simulink model "FMCW_FPGA_Algorithm_Sim"  (R2026a)
settings: Solver=FixedStepDiscrete  StartTime=0  StopTime=simFpgaStopTime  FixedStep=simTs
undefined symbols (not defined in the file): simTemperatureSetpointC, simTs
settings Model: Creator=Administrator  LastModifiedBy=Administrator

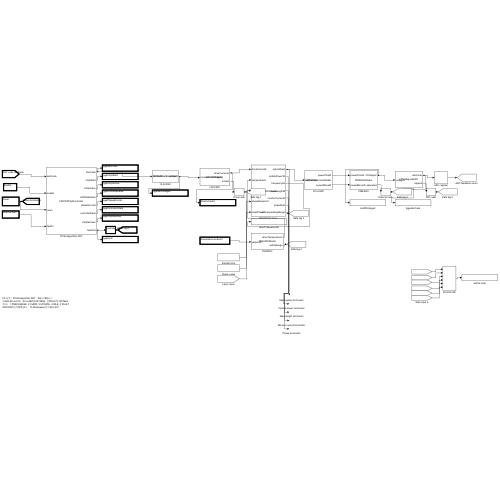
[thumbnail: Simulink's stored preview of the top-level diagram]
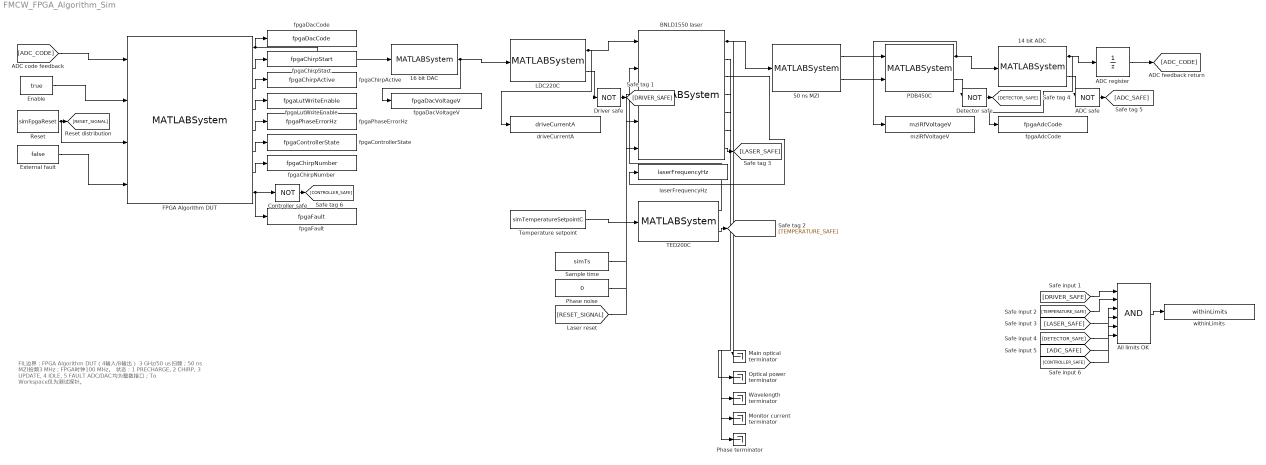
== system FMCW_FPGA_Algorithm_Sim ==
  note: FIL边界：FPGA Algorithm DUT（4输入/8输出）
      | 3 GHz/50 us扫频；50 ns MZI拍频3 MHz；FPGA时钟100 MHz。
      | 状态：1 PRECHARGE, 2 CHIRP, 3 UPDATE, 4 IDLE, 5 FAULT
      | ADC/DAC均为整数接口；To Workspace仅为测试探针。
  14 bit ADC : MATLABSystem  System=FPGASignedADC  Bits=14  FullScaleV=2  SimulateUsing=Code generation
      settings: OpenFcn=open_fmcwlidar_manual('ADC');
      mask Type: FPGASignedADC
  16 bit DAC : MATLABSystem  System=FPGAOffsetBinaryDAC  Bits=16  FullScaleV=2  SimulateUsing=Code generation
      settings: OpenFcn=open_fmcwlidar_manual('DAC');
      mask Type: FPGAOffsetBinaryDAC
  50 ns MZI : MATLABSystem  System=MZIInterferometerModel  SampleTimeS=10e-9  DelayS=50e-9  TapPowerRatio=1e-4  InsertionTransmission=0.90  BiasPhaseRad=0  SimulateUsing=Code generation
      settings: OpenFcn=open_fmcwlidar_manual('MZI');
      mask Type: MZIInterferometerModel
  ADC register : UnitDelay  InitialCondition=int16(0)  SampleTime=simTs
  ADC safe : Logic  Operator=NOT  AllPortsSameDT=off  OutDataTypeStr=boolean
  All limits OK : Logic  Inputs=6  AllPortsSameDT=off  OutDataTypeStr=boolean
  BNLD1550 laser : MATLABSystem  System=BNLD1550Laser  CenterWavelengthM=1550e-9  ReferenceTemperatureC=25  ReferenceCurrentA=650e-3  ThresholdCurrentA=50e-3  MaximumOperatingCurrentA=800e-3  MinimumOperatingTemperatureC=15  MaximumOperatingTemperatureC=35  MaximumModeledPowerW=150e-3  SlopeEfficiencyWPerA=0.25  LinewidthHz=100e3  CurrentTuningHzPerMilliamp=0.3e9  CurrentTuningSign=-1  WavelengthTemperatureCoefficientMPerC=0.1e-9  MonitorResponsivityAPerW=15.5e-3  SimulateUsing=Code generation
      settings: OpenFcn=open_fmcwlidar_manual('BNLD1550');
      mask Type: BNLD1550Laser
  Controller safe : Logic  Operator=NOT  AllPortsSameDT=off  OutDataTypeStr=boolean
  Detector safe : Logic  Operator=NOT  AllPortsSameDT=off  OutDataTypeStr=boolean
  Driver safe : Logic  Operator=NOT  AllPortsSameDT=off  OutDataTypeStr=boolean
  Enable : Constant  Value=true  OutDataTypeStr=boolean
  External fault : Constant  Value=false  OutDataTypeStr=boolean
  FPGA Algorithm DUT : MATLABSystem  System=FMCWFPGAController  ChirpSamples=5000  PrechargeSamples=2000  UpdateSamples=5000  IdleSamples=23000  EdgeSamples=300  DacBits=16  DacFullScaleV=2  BiasCurrentA=650e-3  CurrentGainAPerV=200e-3  ActualDriverBandwidthHz=50e3  SampleTimeS=10e-9  LaserSensitivityHzPerA=-0.3e12  SweepBandwidthHz=3e9  MziDelaySamples=5  NcoStep=uint16( 3 )  LearningNumerator=13  LearningDenominator=20  SimulateUsing=Code generation
      settings: OpenFcn=open_fmcwlidar_manual('FPGA');
      mask Type: FMCWFPGAController
  LDC220C : MATLABSystem  System=LDC220CModel  SampleTimeS=10e-9  BiasCurrentA=650e-3  InitialCurrentA=650e-3  ModulationGainAPerV=206e-3  ModulationBandwidthHz=50e3  CurrentMinA=0  CurrentMaxA=2  ModulationInputMinV=-10  ModulationInputMaxV=10  SimulateUsing=Code generation
      settings: OpenFcn=open_fmcwlidar_manual('LDC220C');
      mask Type: LDC220CModel
  Main optical terminator : Terminator
  Monitor current terminator : Terminator
  Optical power terminator : Terminator
  PDB450C : MATLABSystem  System=PDB450CModel  SampleTimeS=10e-9  Visibility=0.98  ResponsivityAPerW=1.0  LoadedGainVPerA=50e3  BandwidthHz=4e6  OutputSwingV=2.3  DifferentialSaturationW=46e-6  DamagePowerPerDiodeW=20e-3  SimulateUsing=Code generation
      settings: OpenFcn=open_fmcwlidar_manual('PDB450C');
      mask Type: PDB450CModel
  Phase noise : Constant  Value=0
  Phase terminator : Terminator
  Reset : FromWorkspace  VariableName=simFpgaReset  Interpolate=off  OutputAfterFinalValue=Holding final value
  Sample time : Constant  Value=simTs
  TED200C : MATLABSystem  System=TED200CModel  SampleTimeS=10e-9  InitialTemperatureC=25  AmbientTemperatureC=25  ThermalTimeConstantS=2  MinimumSetpointC=15  MaximumSetpointC=35  SimulateUsing=Code generation
      settings: OpenFcn=open_fmcwlidar_manual('TED200C');
      mask Type: TED200CModel
  Temperature setpoint : Constant  Value=simTemperatureSetpointC
  Wavelength terminator : Terminator
  driveCurrentA : ToWorkspace  VariableName=driveCurrentA  SaveFormat=Timeseries  SampleTime=-1
  fpgaAdcCode : ToWorkspace  VariableName=fpgaAdcCode  SaveFormat=Timeseries  SampleTime=-1
  fpgaChirpActive : ToWorkspace  VariableName=fpgaChirpActive  SaveFormat=Timeseries  SampleTime=-1
  fpgaChirpNumber : ToWorkspace  VariableName=fpgaChirpNumber  SaveFormat=Timeseries  SampleTime=-1
  fpgaChirpStart : ToWorkspace  VariableName=fpgaChirpStart  SaveFormat=Timeseries  SampleTime=-1
  fpgaControllerState : ToWorkspace  VariableName=fpgaControllerState  SaveFormat=Timeseries  SampleTime=-1
  fpgaDacCode : ToWorkspace  VariableName=fpgaDacCode  SaveFormat=Timeseries  SampleTime=-1
  fpgaDacVoltageV : ToWorkspace  VariableName=fpgaDacVoltageV  SaveFormat=Timeseries  SampleTime=-1
  fpgaFault : ToWorkspace  VariableName=fpgaFault  SaveFormat=Timeseries  SampleTime=-1
  fpgaLutWriteEnable : ToWorkspace  VariableName=fpgaLutWriteEnable  SaveFormat=Timeseries  SampleTime=-1
  fpgaPhaseErrorHz : ToWorkspace  VariableName=fpgaPhaseErrorHz  SaveFormat=Timeseries  SampleTime=-1
  laserFrequencyHz : ToWorkspace  VariableName=laserFrequencyHz  SaveFormat=Timeseries  SampleTime=-1
  mziRfVoltageV : ToWorkspace  VariableName=mziRfVoltageV  SaveFormat=Timeseries  SampleTime=-1
  withinLimits : ToWorkspace  VariableName=withinLimits  SaveFormat=Timeseries  SampleTime=-1
  wires:
  [ADC_CODE] -> FPGA Algorithm DUT/1
  Enable/1 -> FPGA Algorithm DUT/2
  Reset/1 -> FPGA Algorithm DUT/3, [RESET_SIGNAL]
  External fault/1 -> FPGA Algorithm DUT/4
  FPGA Algorithm DUT/1 -> 16 bit DAC/1, fpgaDacCode/1
  16 bit DAC/1 -> LDC220C/1, fpgaDacVoltageV/1
  LDC220C/1 -> BNLD1550 laser/1, driveCurrentA/1
  Temperature setpoint/1 -> TED200C/1
  TED200C/1 -> BNLD1550 laser/2
  Sample time/1 -> BNLD1550 laser/3
  Phase noise/1 -> BNLD1550 laser/4
  [RESET_SIGNAL] -> BNLD1550 laser/5
  BNLD1550 laser/1 -> 50 ns MZI/1, Main optical terminator/1
  50 ns MZI/1 -> PDB450C/1
  50 ns MZI/2 -> PDB450C/2
  PDB450C/1 -> 14 bit ADC/1, mziRfVoltageV/1
  14 bit ADC/1 -> ADC register/1, fpgaAdcCode/1
  ADC register/1 -> [ADC_CODE]
  BNLD1550 laser/2 -> Optical power terminator/1
  BNLD1550 laser/4 -> Wavelength terminator/1
  BNLD1550 laser/5 -> Monitor current terminator/1
  BNLD1550 laser/6 -> Phase terminator/1
  LDC220C/2 -> Driver safe/1
  PDB450C/2 -> Detector safe/1
  14 bit ADC/2 -> ADC safe/1
  FPGA Algorithm DUT/8 -> Controller safe/1, fpgaFault/1
  Driver safe/1 -> [DRIVER_SAFE]
  TED200C/2 -> [TEMPERATURE_SAFE]
  BNLD1550 laser/7 -> [LASER_SAFE]
  Detector safe/1 -> [DETECTOR_SAFE]
  ADC safe/1 -> [ADC_SAFE]
  Controller safe/1 -> [CONTROLLER_SAFE]
  [DRIVER_SAFE] -> All limits OK/1
  [TEMPERATURE_SAFE] -> All limits OK/2
  [LASER_SAFE] -> All limits OK/3
  [DETECTOR_SAFE] -> All limits OK/4
  [ADC_SAFE] -> All limits OK/5
  [CONTROLLER_SAFE] -> All limits OK/6
  FPGA Algorithm DUT/2 -> fpgaChirpStart/1
  FPGA Algorithm DUT/3 -> fpgaChirpActive/1
  FPGA Algorithm DUT/4 -> fpgaLutWriteEnable/1
  FPGA Algorithm DUT/5 -> fpgaPhaseErrorHz/1
  FPGA Algorithm DUT/6 -> fpgaControllerState/1
  FPGA Algorithm DUT/7 -> fpgaChirpNumber/1
  BNLD1550 laser/3 -> laserFrequencyHz/1
  All limits OK/1 -> withinLimits/1
